simulink model "Serial_Receive"  (R2025b)
settings: Solver=FixedStepAuto  StartTime=0.0  StopTime=100  FixedStep=0.01  RelTol=1e-3
libraries: instrumentseriallib x2
settings Model: ExtModeTrigDuration=2  Creator=CoolA  LastModifiedBy=CoolA
settings SolverCC: AutoInsertRateTranBlk=on
settings OptimizationCC: EnhancedBackFolding=on  PassReuseOutputArgsAs=Individual arguments  ZeroExternalMemoryAtStartup=off  ZeroInternalMemoryAtStartup=off  MaxStackSize=64  OptimizeBlockOrder=speed  DifferentSizesBufferReuse=on  OptimizationCustomize=off  EfficientTunableParamExpr=on
settings DebuggingCC: ParameterTunabilityLossMsg=error
settings HardwareCC: ProdBitPerInt=16.0  ProdBitPerPointer=16.0  ProdBitPerSizeT=16.0  ProdBitPerPtrDiffT=16.0  ProdLargestAtomicFloat=None  ProdWordSize=8.0  ProdHWDeviceType=Atmel->AVR  UseEmbeddedCoderFeatures=off  UseSimulinkCoderFeatures=off
settings RTWCC: SystemTargetFile=ert.tlc  HardwareBoard=Arduino Uno  TemplateMakefile=ert_default_tmf  Toolchain=Arduino AVR  Description=Embedded Coder
settings CodeAppCC: ForceParamTrailComments=on  IgnoreCustomStorageClasses=off  OperatorAnnotations=on  SimulinkDataObjDesc=on  SFDataObjDesc=on  InsertBlockDesc=on
settings ERTTargetCC: ExtModeTransport=3.0  ExtModeStaticAlloc=on  ExtModeAutomaticAllocSize=off  ExtModeStaticAllocSize=250.0  ExtModeMexFile=ext_xcp  ExtModeIntrfLevel=Level2 - Open  InlinedParameterPlacement=Hierarchical  SupportContinuousTime=on  SupportNonInlinedSFcns=on  SupportVariableSizeSignals=on

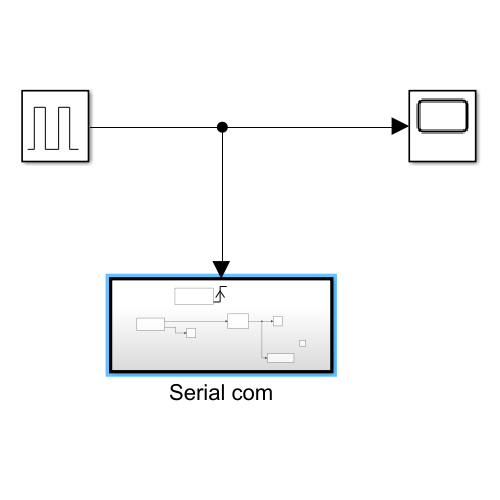
[thumbnail: Simulink's stored preview of the top-level diagram]
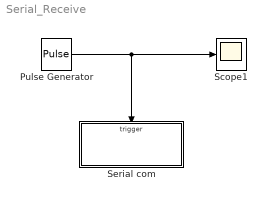
== system Serial_Receive ==
  Pulse Generator : DiscretePulseGenerator  PulseType=Time based  Period=0.02  PulseWidth=50
  Scope1 : Scope
      settings: ActiveDisplayYMinimum=-1  ActiveDisplayYMaximum=1
  Serial com : Subsystem  TreatAsAtomicUnit=on
  wires:
  Pulse Generator/1 -> Scope1/1, Serial com/Trigger

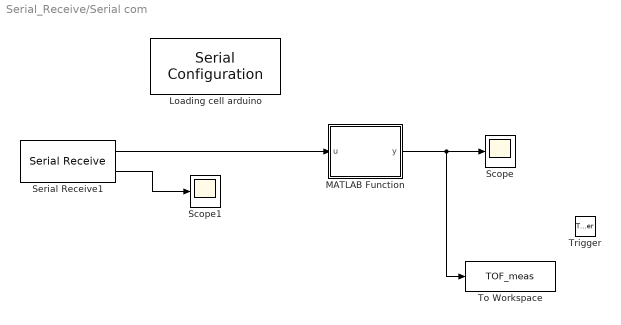
== system Serial_Receive/Serial com ==
  Trigger : TriggerPort  VariantControl=(inherit)
  Loading cell arduino : instrumentseriallib/Serial Configuration  Priority=-200000  PortSel=COM3  Port=COM3  ComPort=COM3  BaudRate=115200  DataBits=8  Parity=none  StopBits=1  ByteOrder=little-endian  FlowControl=none  Timeout=10  SimulateUsing=Interpreted execution  BlockInModel=on  aMode=1
  MATLAB Function : MATLAB Function  TreatAsAtomicUnit=on
  Scope : Scope
      settings: ActiveDisplayYMinimum=-3015.125  ActiveDisplayYMaximum=2906.125  DataLoggingVariableName=ScopeData6
  Scope1 : Scope
      settings: ActiveDisplayYMinimum=-0.12499999999999997  ActiveDisplayYMaximum=1.125  DataLoggingVariableName=ScopeData7
  Serial Receive1 : instrumentseriallib/Serial Receive  Priority=1  PortSel=COM3  Port=COM3  ComPort=COM3  DataType=uint8  SaveDataType=uint8  ToggleHeader=off  Header=[]  ToggleDataSize=on  DataSize=[6 1]  ToggleTerminator=off  Terminator=<none>  CustomTerminator=[]  InputFormat=Column major  EnableBlockingMode=off  ActionDataUnavailable=Output last received value  ActionWhenDataUnavailable=Output last received value  CustomValue=0  SampleTime=-1  SimulateUsing=Interpreted execution  BlockInModel=on  aMode=1  LibraryInUse=instrumentlib
  To Workspace : ToWorkspace  VariableName=TOF_meas  SaveFormat=Timeseries  SampleTime=-1
  wires:
  Serial Receive1/1 -> MATLAB Function/1(u)
  MATLAB Function/1(y) -> To Workspace/1, Scope/1
  Serial Receive1/2 -> Scope1/1

== matlab function Serial_Receive/Serial com/MATLAB Function ==
  data: u input; y output size=[7 1]
function y = parseSerial(u)

persistent buffer
persistent previous_output

if isempty(previous_output)
    previous_output = 0;
end

if isempty(buffer)
    buffer = '';
end

% Append new data
buffer = [buffer char(u')];

y = previous_output;  % default output

while true
    
    startIdx = strfind(buffer, '<');
    endIdx   = strfind(buffer, '>');
    
    % Need both markers
    if isempty(startIdx) || isempty(endIdx)
        y = previous_output;
        break;
    end
    
    % Case 1: end comes before start → discard garbage
    if endIdx(1) < startIdx(1)
        buffer = buffer(endIdx(1)+1:end);
        continue;
    end
    
    % Case 2: valid packet exists
    if startIdx(1) < endIdx(1)
        
        msg = buffer(startIdx(1)+1 : endIdx(1)-1);
        %disp(msg)
        
        % Remove processed part
        buffer = buffer(endIdx(1)+1:end);
        
        vals = sscanf(msg, '%f,%f,%f,%f,%f,%f,%f');
        
        if isscalar(vals)
            y = 0;
            y(:) = vals;  
            previous_output = y;
            return;   % exit after one valid packet
        end
    end
end
